simulink model "LINEALIZACIONPLANTAPROmac2"  (R2021a)
settings: Solver=ode45  StartTime=0.0  StopTime=10  RelTol=1e-3
values from neighbouring files (symbols this model uses):
  b = 0.00014    [Parametros_Modelo.m]
  f = 60    [Parametros_Modelo.m]
  Freq = 100    [Parametros_Modelo.m]
  Lm = 0.0117    [Parametros_Modelo.m]
  Lr = 0.014    [Parametros_Modelo.m]
  Ls = 0.014    [Parametros_Modelo.m]
  p = 4    [Parametros_Modelo.m]
  Rr = 3.9    [Parametros_Modelo.m]
  Rs = 1.7    [Parametros_Modelo.m]
undefined symbols (not defined in the file or in its folder): H
settings Model: Creator=electronica  LastModifiedBy=hubertdelgado
settings DebuggingCC: UnconnectedInputMsg=none  UnconnectedOutputMsg=none  UnconnectedLineMsg=none
settings ModelReferenceCC: EnableRefExpFcnMdlSchedulingChecks=off
settings RTWCC: Description=Generic Real-Time Target  DLArmComputeVersion=20.02.1

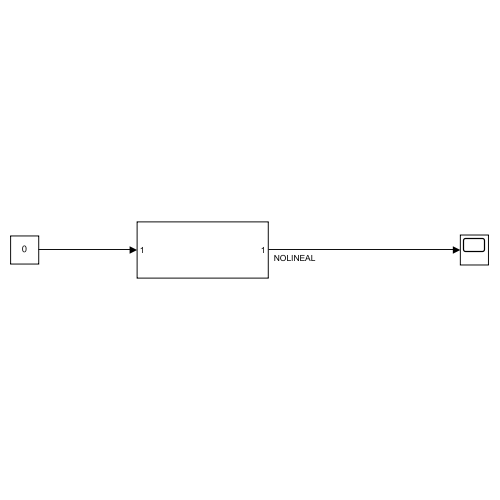
[thumbnail: Simulink's stored preview of the top-level diagram]
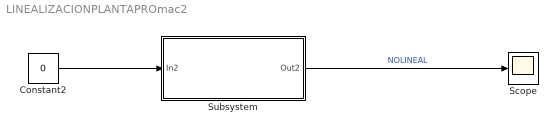
== system LINEALIZACIONPLANTAPROmac2 ==
  Constant2 : Constant  Value=0
  Scope : Scope
  Subsystem : Subsystem
  wires:
  Constant2/1 -> Subsystem/1(In2)
  Subsystem/1(Out2) -> Scope/1  "NOLINEAL"

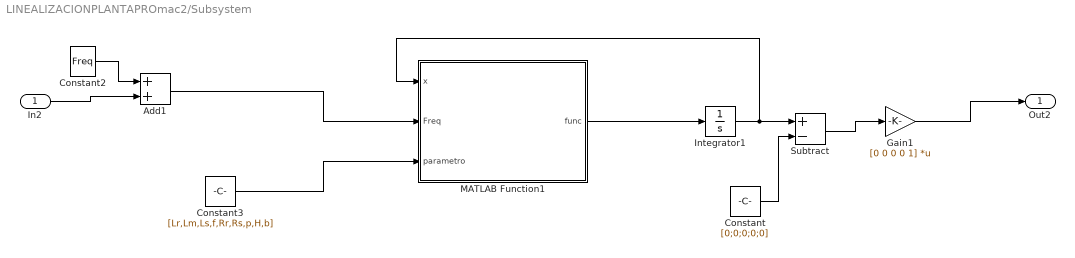
== system LINEALIZACIONPLANTAPROmac2/Subsystem ==
  In2 : Inport
  Add1 : Sum
  Constant : Constant  Value=[0;0;0;0;0]
  Constant2 : Constant  Value=Freq
  Constant3 : Constant  Value=[Lr,Lm,Ls,f,Rr,Rs,p,H,b]
  Gain1 : Gain  Gain=[0 0 0 0 1]  Multiplication=Matrix(K*u)
  Integrator1 : Integrator  InitialCondition=[0;0;0;0;0]
  MATLAB Function1 : MATLAB Function  TreatAsAtomicUnit=on
  Subtract : Sum  Inputs=+-
  Out2 : Outport
  wires:
  Add1/1 -> MATLAB Function1/2(Freq)
  Integrator1/1 -> Subtract/1, MATLAB Function1/1(x)
  Constant3/1 -> MATLAB Function1/3(parametro)
  MATLAB Function1/1(func) -> Integrator1/1
  Gain1/1 -> Out2/1
  Constant2/1 -> Add1/1
  In2/1 -> Add1/2
  Subtract/1 -> Gain1/1
  Constant/1 -> Subtract/2

== matlab function LINEALIZACIONPLANTAPROmac2/Subsystem/MATLAB Function1 ==
  data: x input; func output; Freq input; parametro input
function func = fcn(x,Freq,parametro)
%Parametros
Lr = parametro(1);
Lm = parametro(2);
Ls = parametro(3);
f = parametro(4);
Rr = parametro(5);
Rs = parametro(6);
p = parametro(7);
H = parametro(8);
b = parametro(9);

%Estados
Ids = x(1);
Iqs = x(2);
Idr = x(3);
Iqr = x(4);
wm = x(5);

delta = (Lr+Lm)*(Ls+Lm)-Lm^2;
ws = 2*pi*f;
R = [Rs 0 0 0;
      0 Rs 0 0;
      0 0 Rr 0;
      0 0 0 Rr];

omega = [0, -ws, 0, 0;
    ws, 0, 0, 0;
    0, 0, 0, -(ws-(p*wm/2));
    0, 0, (ws-(p*wm/2)), 0];


L = [Ls+Lm, 0, Lm, 0;
    0, Ls+Lm 0, Lm;
    Lm, 0, Lr+Lm, 0;
    0, Lm, 0, Lr+Lm];

inv_L = (1/delta)*[Lr+Lm, 0, -Lm, 0;
                  0, Lr+Lm, 0, -Lm;
                  -Lm, 0, Ls+Lm, 0;
                  0, -Lm, 0, Ls+Lm];

Vqs = Freq;
V = [0;
       Vqs;
       0;
       0];

I = [Ids;
    Iqs;
    Idr;
    Iqr];

dI = -(inv_L*R + inv_L*omega*L)*I + inv_L*V;
Te = 1.5*p*Lm*(Iqs*Idr - Ids*Iqr);
dwm = (p/H)*(Te - (b/H)*wm);
func = [dI; dwm];
